simulink model "q3labo2finalclement"  (R2016a)
settings: Solver=VariableStepAuto  StartTime=0.0  StopTime=10.0  RelTol=1e-3
values from neighbouring files (symbols this model uses):
  a_equa1 = a(1)*sqrt(1-((L)*H)/T(1))    [labo2 - clement.m]    (also in labo2 - merge-q1q2.m; labo2-part1FINAL.m; labo2finalclement.m)
  a_equa2 = a    [labo2 - clement.m]    (also in labo2 - merge-q1q2.m; labo2-part1FINAL.m; labo2finalclement.m)
  H = [0:1000:20000]    [labo2 - clement.m]    (also in labo2 - merge-q1q2.m; labo2-part1FINAL.m; labo2finalclement.m)
  k = 1.4    [labo2finalclement.m]
  M = [0:0.2:2]    [lab2raf.m]    (also in labo2 - merge-q1q2.m; labo2-part1FINAL.m; labo2finalclement.m)
  P_equa1 = P(1)*(1-((L)*H)/T(1)).^((g0)/(L*R))    [labo2 - clement.m]    (also in labo2 - merge-q1q2.m; labo2-part1FINAL.m; labo2finalclement.m)
  P_equa2 = P(1)*exp((-g0./(R*T)).*(H-H(1)))    [labo2 - clement.m]    (also in labo2 - merge-q1q2.m; labo2-part1FINAL.m; labo2finalclement.m)
  PtPsM = cat(2, PtPsM1, PtPsM2)    [lab2raf.m]    (also in labo2 - merge-q1q2.m; labo2-part1FINAL.m; labo2finalclement.m)
  Qc = zeros(1,size(Vc,2))    [labo2 - clement.m]    (also in labo2 - merge-q1q2.m; labo2-part1FINAL.m; labo2finalclement.m)
  R = 287    [labo2 - clement.m]    (also in labo2 - merge-q1q2.m; labo2-part1FINAL.m; labo2finalclement.m)
  rho_equa1 = rho(1)*(1-((L)*H)/T(1)).^(((g0)/(L*R))-1)    [labo2 - clement.m]    (also in labo2 - merge-q1q2.m; labo2-part1FINAL.m; labo2finalclement.m)
  rho_equa2 = rho(1)*exp((-g0./(R*T)).*(H-H(1)))    [labo2 - clement.m]    (also in labo2 - merge-q1q2.m; labo2-part1FINAL.m; labo2finalclement.m)
  T_equa1 = T(1)*(1-((L)*H)/T(1))    [labo2 - clement.m]    (also in labo2 - merge-q1q2.m; labo2-part1FINAL.m; labo2finalclement.m)
  T_equa2 = T    [labo2 - clement.m]    (also in labo2 - merge-q1q2.m; labo2-part1FINAL.m; labo2finalclement.m)
  Vc = [0:10:600]    [labo2 - clement.m]    (also in labo2 - merge-q1q2.m; labo2-part1FINAL.m; labo2finalclement.m)
undefined symbols (not defined in the file or in its folder): index, Psort
libraries: simulink x2, aerolibconvert2 x1
settings Model: Creator=Clément  LastModifiedBy=Clément

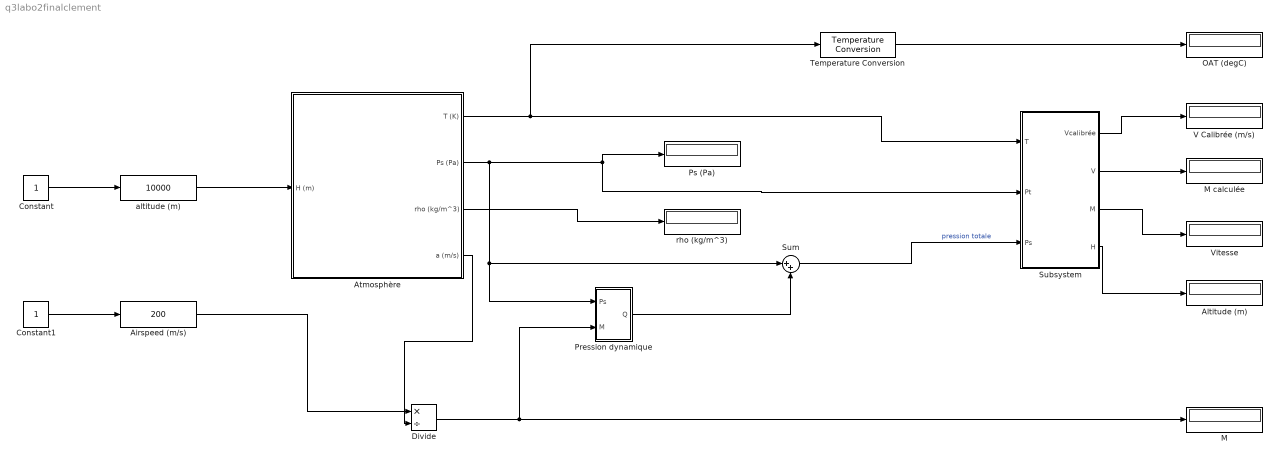
== system q3labo2finalclement ==
  Airspeed (m/s) : simulink/Math Operations/Slider Gain  low=0  gain=200  high=500
  Altitude (m) : Display
      settings: Decimation=50
  Atmosphère : Subsystem
  Constant : Constant
  Constant1 : Constant
  Divide : Product  Inputs=*/
  M : Display
      settings: Decimation=50
  M calculée : Display
      settings: Decimation=50
  OAT (degC) : Display
      settings: Decimation=50
  Pression dynamique : Subsystem
  Ps (Pa) : Display
      settings: Decimation=50
  Subsystem : Subsystem
  Sum : Sum  Inputs=|++
  Temperature Conversion : aerolibconvert2/Temperature Conversion  IU=K  OU=C
  V Calibrée (m/s) : Display
      settings: Decimation=50
  Vitesse : Display
      settings: Decimation=50
  altitude (m) : simulink/Math Operations/Slider Gain  low=0  gain=10000  high=30000
  rho (kg/m^3) : Display
      settings: Decimation=50
  wires:
  Constant/1 -> altitude (m)/1
  Constant1/1 -> Airspeed (m/s)/1
  Temperature Conversion/1 -> OAT (degC)/1
  Airspeed (m/s)/1 -> Divide/1
  Divide/1 -> Pression dynamique/2(M), M/1
  altitude (m)/1 -> Atmosphère/1(H (m))
  Atmosphère/1(T (K)) -> Subsystem/1(T), Temperature Conversion/1
  Atmosphère/4(a (m/s)) -> Divide/2
  Atmosphère/2(Ps (Pa)) -> Pression dynamique/1(Ps), Sum/1, Subsystem/2(Pt), Ps (Pa)/1
  Atmosphère/3(rho (kg/m^3)) -> rho (kg/m^3)/1
  Pression dynamique/1(Q) -> Sum/2
  Sum/1 -> Subsystem/3(Ps)  "pression totale"
  Subsystem/1(Vcalibrée) -> V Calibrée (m/s)/1
  Subsystem/2(V) -> M calculée/1
  Subsystem/3(M) -> Vitesse/1
  Subsystem/4(H) -> Altitude (m)/1

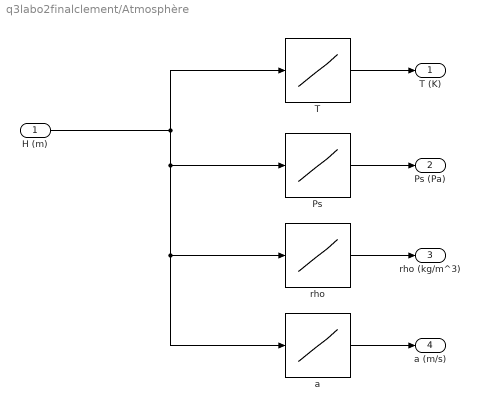
== system q3labo2finalclement/Atmosphère ==
  H (m) : Inport
  Ps : Lookup_n-D  NumberOfTableDimensions=1  BreakpointsForDimension1=H  Table=[P_equa1 P_equa2]  InternalRulePriority=Speed  RndMeth=Simplest  InputSameDT=on
  T : Lookup_n-D  NumberOfTableDimensions=1  BreakpointsForDimension1=H  Table=[T_equa1 T_equa2]  InternalRulePriority=Speed  RndMeth=Simplest  InputSameDT=on
  a : Lookup_n-D  NumberOfTableDimensions=1  BreakpointsForDimension1=H  Table=[a_equa1 a_equa2]  InternalRulePriority=Speed  RndMeth=Simplest  InputSameDT=on
  rho : Lookup_n-D  NumberOfTableDimensions=1  BreakpointsForDimension1=H  Table=[rho_equa1 rho_equa2]  InternalRulePriority=Speed  RndMeth=Simplest  InputSameDT=on
  T (K) : Outport
  Ps (Pa) : Outport  Port=2
  rho (kg/m^3) : Outport  Port=3
  a (m/s) : Outport  Port=4
  wires:
  H (m)/1 -> T/1, a/1, rho/1, Ps/1
  T/1 -> T (K)/1
  Ps/1 -> Ps (Pa)/1
  rho/1 -> rho (kg/m^3)/1
  a/1 -> a (m/s)/1

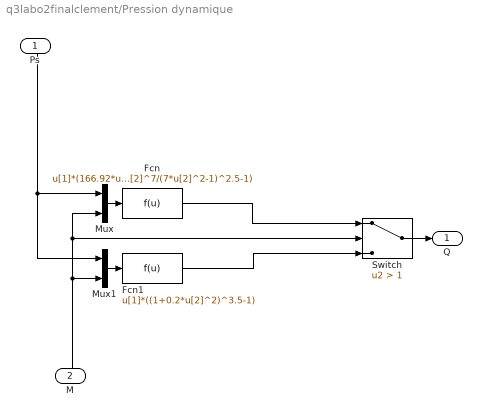
== system q3labo2finalclement/Pression dynamique ==
  Ps : Inport
  M : Inport  Port=2
  Fcn : Fcn  Expr=u[1]*(166.92*u[2]^7/(7*u[2]^2-1)^2.5-1)
  Fcn1 : Fcn  Expr=u[1]*((1+0.2*u[2]^2)^3.5-1)
  Mux : Mux  Inputs=2
  Mux1 : Mux  Inputs=2
  Switch : Switch  Criteria=u2 > Threshold  Threshold=1
  Q : Outport
  wires:
  Fcn/1 -> Switch/1
  M/1 -> Mux/2, Switch/2, Mux1/2
  Ps/1 -> Mux1/1, Mux/1
  Switch/1 -> Q/1
  Mux1/1 -> Fcn1/1
  Fcn1/1 -> Switch/3
  Mux/1 -> Fcn/1

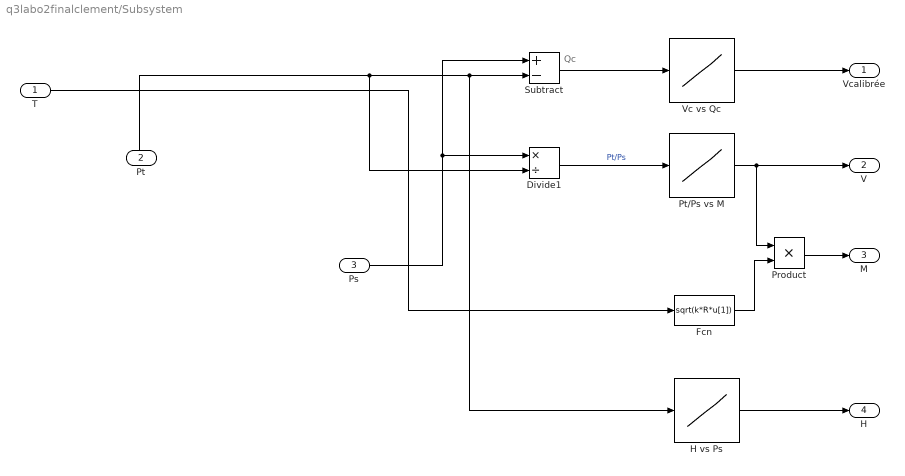
== system q3labo2finalclement/Subsystem ==
  note: Qc
  T : Inport
  Pt : Inport  Port=2
  Ps : Inport  Port=3
  Divide1 : Product  Inputs=*/
  Fcn : Fcn  Expr=sqrt(k*R*u[1])
  H vs Ps : Lookup_n-D  NumberOfTableDimensions=1  BreakpointsForDimension1=Psort  Table=H(index)  InternalRulePriority=Speed  RndMeth=Simplest  InputSameDT=on
  Product : Product
  Pt/Ps vs M : Lookup_n-D  NumberOfTableDimensions=1  BreakpointsForDimension1=PtPsM  Table=M  InternalRulePriority=Speed  RndMeth=Simplest  InputSameDT=on
  Subtract : Sum  Inputs=+-
  Vc vs Qc : Lookup_n-D  NumberOfTableDimensions=1  BreakpointsForDimension1=Qc  Table=Vc  InternalRulePriority=Speed  RndMeth=Simplest  InputSameDT=on
  Vcalibrée : Outport
  V : Outport  Port=2
  M : Outport  Port=3
  H : Outport  Port=4
  wires:
  Vc vs Qc/1 -> Vcalibrée/1
  Pt/1 -> Divide1/2, H vs Ps/1, Subtract/2
  T/1 -> Fcn/1
  Ps/1 -> Subtract/1, Divide1/1
  Subtract/1 -> Vc vs Qc/1
  Pt/Ps vs M/1 -> V/1, Product/1
  Fcn/1 -> Product/2
  Product/1 -> M/1
  H vs Ps/1 -> H/1
  Divide1/1 -> Pt/Ps vs M/1  "Pt/Ps"
